simulink model "Commando07012014withscope"  (R2012b)
settings: Solver=ode5  StartTime=0.0  StopTime=inf  FixedStep=sample_time  RelTol=1e-3
InitFcn:
  | sample_time=0.005;%0.004;%0.0025;%0.02;
  | sample_time_Vicon = 0.005;
  | DeltaT = 0.02;
  | g = 9.81;
  | H0 = g%0.3165;
  | Kl = 1;
  | 
  | Q6_mass = 0.8;
  | 
  | Q6_Omega_r = 1.2; %for horizon ref
  | Q6_Zeta_r = 0.707; %for horizon ref
  | Q6_Omega_r_h = 2;%for vertical ref
  | Q6_Zeta_r_h = 0.7; %for vertical ref
  | 
  | 
  | Q6_Omega = 1.5; %for horizon control
  | Q6_Zeta = 0.507; %for horizon control
  | Q6_Omega_h= 2; %for vertical control
  | Q6_Zeta_h = 0.5; %for vertical control
  | 
  | 
  | Q6_acc_max = 5;%horizontal max acc
  | Q6_acc_max_h = 5;%horizontal max acc
  | 
  | omega_circle = 20*pi/180;
  | 
  | omega_h = 0.1;%Ascending speed
  | PI = pi;
  | Circle_R = 1.9;
  | 
  | 
  | MAX_Height = -2;
  | 
  | 
  | % for NN
  | n = 5;
  | r = 3;
  | n2 = 5;
  | NN_ST = 0.02;
  | 
  | GAMA_V = 6;
  | gama_V_e = 0.01;
  | 
  | GAMA_W = GAMA_V;
  | gama_W_e =0.01;
  | 
  | % deadzone
  | NN_Deadzone_Z = 0;
  | 
  | % inputs nomalizaton parameters
  | NN_Z_y_min = -3;
  | NN_Z_y_max = 0.5;
  | 
  | NN_Z_v_max = 8;
  | NN_Z_v_min = -NN_Z_v_max;
  | 
  | % alpha = 0.034;
  | alpha = 1;
  | % c_f = 0.0015;
  | c_f = 0.001;
  | ... (+1 lines)
libraries: X330_Control x20, simulink x10
(part 2 of 2)

== stateflow chart Commando07012014withscope/Subsystem/Trajectory Logic/ SF ==
  state Airborne
    state TakeOff
      du:		HoverThrottle = (H0 - HoverThrottle)*2*DeltaT + HoverThrottle ;
      PosDes_UAV1[2] = (-1.2 - PosDes_UAV1[2])*1*DeltaT + PosDes_UAV1[2] ;
      PosDes_UAV2[2] = (-1.2 - PosDes_UAV2[2])*1*DeltaT + PosDes_UAV2[2] ;
      PosDes_UAV3[2] = (-1.2 - PosDes_UAV3[2])*1*DeltaT + PosDes_UAV3[2] ;
      PosDes_UAV4[2] = (-1.2 - PosDes_UAV4[2])*1*DeltaT + PosDes_UAV4[2] ;
    state StartPoint
      state StartPoint_UAV1 [parallel]
        du:PosDes_UAV1[0] = (Circle_R*sin(0*PI/180 )- PosDes_UAV1[0])*1*DeltaT + PosDes_UAV1[0] ;
        PosDes_UAV1[1] = (Circle_R*cos(0*PI/180 )- PosDes_UAV1[1])*1*DeltaT + PosDes_UAV1[1] ;
        settings: executionOrder=1
      state StartPoint_UAV2 [parallel]
        du:PosDes_UAV2[0] = (Circle_R*sin(90*PI/180)-PosDes_UAV2[0])*0.5*DeltaT+PosDes_UAV2[0];
        PosDes_UAV2[1] = (Circle_R*cos(90*PI/180)-PosDes_UAV2[1])*0.5*DeltaT+PosDes_UAV2[1];
        settings: executionOrder=2
      state StartPoint_UAV3 [parallel]
        du:PosDes_UAV3[0] = (Circle_R*sin(180*PI/180)-PosDes_UAV3[0])*1*DeltaT + PosDes_UAV3[0];
        PosDes_UAV3[1] = (Circle_R*cos(180*PI/180)-PosDes_UAV3[1])*1*DeltaT+PosDes_UAV3[1];
        settings: executionOrder=3
      state test [parallel]
        settings: executionOrder=4
        state StartPoint_UAV4
          du:PosDes_UAV4[0] = (Circle_R*sin(270*PI/180)-PosDes_UAV4[0])*1*DeltaT+PosDes_UAV4[0];
          PosDes_UAV4[1] = (Circle_R*cos(270*PI/180)-PosDes_UAV4[1])*1*DeltaT+PosDes_UAV4[1];
        state Null
        (default) -> Null
        Null -> StartPoint_UAV4 : after(2,sec)
    state flyingcircle
      state Circle2D [parallel]
        du: PosDes_UAV1[0] = Circle_R*sin(0*PI/180 + T_circle*omega_circle);
        PosDes_UAV1[1] = Circle_R*cos(0*PI/180 + T_circle*omega_circle);
        PosDes_UAV1[2]= Pos_UAV5[2]-0.2;
        settings: executionOrder=1
      state Circle2D3 [parallel]
        du: PosDes_UAV4[0] = Circle_R*sin(270*PI/180 + T_circle*omega_circle);
        PosDes_UAV4[1] = Circle_R*cos(270*PI/180 + T_circle*omega_circle);
        PosDes_UAV4[2]= Pos_UAV5[2]-0.2;
        settings: executionOrder=2
      state Circle2D1 [parallel]
        du: PosDes_UAV2[0] = Circle_R*sin(90*PI/180 + T_circle*omega_circle);
        PosDes_UAV2[1] = Circle_R*cos(90*PI/180 + T_circle*omega_circle);
        PosDes_UAV2[2]= Pos_UAV5[2]-0.2;
        settings: executionOrder=3
      state T_Incr [parallel]
        du:   T_circle = T_circle + DeltaT;
        settings: executionOrder=4
      state Circle2D2 [parallel]
        du: PosDes_UAV3[0] = Circle_R*sin(180*PI/180 + T_circle*omega_circle);
        PosDes_UAV3[1] = Circle_R*cos(180*PI/180 + T_circle*omega_circle);
        PosDes_UAV3[2]= Pos_UAV5[2]-0.2;
        settings: executionOrder=5
    state flyingcircle1
      du:
      PosDes_UAV1[2] = (-2.7 - PosDes_UAV1[2])*0.5*DeltaT + PosDes_UAV1[2] ;
      PosDes_UAV2[2] = (-2.7 - PosDes_UAV2[2])*0.5*DeltaT + PosDes_UAV2[2] ;
      PosDes_UAV3[2] = (-2.7 - PosDes_UAV3[2])*0.5*DeltaT + PosDes_UAV3[2] ;
      PosDes_UAV4[2] = (-2.7 - PosDes_UAV4[2])*0.5*DeltaT + PosDes_UAV4[2] ;
    state flyingcircle2
      du:
      PosDes_UAV1[2] = (-1.2 - PosDes_UAV1[2])*1*DeltaT + PosDes_UAV1[2] ;
      PosDes_UAV2[2] = (-1.7 - PosDes_UAV2[2])*1*DeltaT + PosDes_UAV2[2] ;
      PosDes_UAV3[2] = (-2.2 - PosDes_UAV3[2])*1*DeltaT + PosDes_UAV3[2] ;
      PosDes_UAV4[2] = (-2.7 - PosDes_UAV4[2])*1*DeltaT + PosDes_UAV4[2] ;
    state endPoints
      du:
      PosDes_UAV1[2] = (-1.0 - PosDes_UAV1[2])*0.5*DeltaT + PosDes_UAV1[2] ;
      PosDes_UAV1[0]=(-2.0-PosDes_UAV1[0])*0.5*DeltaT+PosDes_UAV1[0];
      PosDes_UAV1[1]=(1.5-PosDes_UAV1[1])*0.5*DeltaT+PosDes_UAV1[1];
      PosDes_UAV2[2] = (-1.5 - PosDes_UAV2[2])*0.5*DeltaT + PosDes_UAV2[2] ;
      PosDes_UAV2[0]=(-2.0-PosDes_UAV2[0])*0.5*DeltaT+PosDes_UAV2[0];
      PosDes_UAV2[1]=(0.0-PosDes_UAV2[1])*0.5*DeltaT+PosDes_UAV2[1];
      PosDes_UAV3[2] = (-2.0 - PosDes_UAV3[2])*0.5*DeltaT + PosDes_UAV3[2] ;
      PosDes_UAV3[0]=(-2.0-PosDes_UAV3[0])*0.5*DeltaT+PosDes_UAV3[0];
      PosDes_UAV3[1]=(-1.5-PosDes_UAV3[1])*0.5*DeltaT+PosDes_UAV3[1];
      PosDes_UAV4[2] = (-2.5 - PosDes_UAV4[2])*0.5*DeltaT + PosDes_UAV4[2] ;
      PosDes_UAV4[0]=(-2.0-PosDes_UAV4[0])*0.5*DeltaT+PosDes_UAV4[0];
      PosDes_UAV4[1]=(-3.0-PosDes_UAV4[1])*0.5*DeltaT+PosDes_UAV4[1];
    state endPoints1
      du:
      PosDes_UAV1[2] = (-1.0 - PosDes_UAV1[2])*0.5*DeltaT + PosDes_UAV1[2] ;
      PosDes_UAV1[0]=(-2.0-PosDes_UAV1[0])*0.5*DeltaT+PosDes_UAV1[0];
      PosDes_UAV1[1]=(1.5-PosDes_UAV1[1])*0.5*DeltaT+PosDes_UAV1[1];
      PosDes_UAV2[2] = (-1.0 - PosDes_UAV2[2])*0.5*DeltaT + PosDes_UAV2[2] ;
      PosDes_UAV2[0]=(-2.0-PosDes_UAV2[0])*0.5*DeltaT+PosDes_UAV2[0];
      PosDes_UAV2[1]=(0.0-PosDes_UAV2[1])*0.5*DeltaT+PosDes_UAV2[1];
      PosDes_UAV3[2] = (-1.0 - PosDes_UAV3[2])*0.5*DeltaT + PosDes_UAV3[2] ;
      PosDes_UAV3[0]=(-2.0-PosDes_UAV3[0])*0.5*DeltaT+PosDes_UAV3[0];
      PosDes_UAV3[1]=(-1.5-PosDes_UAV3[1])*0.5*DeltaT+PosDes_UAV3[1];
      PosDes_UAV4[2] = (-1.0 - PosDes_UAV4[2])*0.5*DeltaT + PosDes_UAV4[2] ;
      PosDes_UAV4[0]=(-2.0-PosDes_UAV4[0])*0.5*DeltaT+PosDes_UAV4[0];
      PosDes_UAV4[1]=(-3.0-PosDes_UAV4[1])*0.5*DeltaT+PosDes_UAV4[1];
    (default) -> TakeOff : {	PosDes_UAV1 = Pos_UAV1;
        | 	PosDes_UAV2 = Pos_UAV2;
        | 	PosDes_UAV3 = Pos_UAV3;
        | 	PosDes_UAV4 = Pos_UAV4; }
    TakeOff -> StartPoint : after(3,sec)
    StartPoint -> flyingcircle : [abs(Pos_UAV4[0]-(-2))+abs(Pos_UAV4[1])<0.2]
        | {T_circle = 0.0, Light = 1;}
    flyingcircle -> flyingcircle1 : [RC[5]>0.5]
        | {Light=0;}
    flyingcircle1 -> flyingcircle2 : [abs(Pos_UAV5[0]-(-1))+abs(Pos_UAV5[1]-3.3)<0.3]
    flyingcircle2 -> endPoints : after (3,sec)
    endPoints -> endPoints1 : after (3,sec)
  state Landing
    state Decsending
      en:		PosDes_UAV1 = Pos_UAV1;	PosDes_UAV2 = Pos_UAV2;  PosDes_UAV3 = Pos_UAV3;
      PosDes_UAV4 = Pos_UAV4;
      du:		PosDes_UAV1[2] = (0 - PosDes_UAV1[2])*0.25*DeltaT + PosDes_UAV1[2] ;
      PosDes_UAV2[2] = (0 - PosDes_UAV2[2])*0.25*DeltaT + PosDes_UAV2[2] ;
      PosDes_UAV3[2] = (0 - PosDes_UAV3[2])*0.25*DeltaT + PosDes_UAV3[2] ;
      PosDes_UAV4[2] = (0 - PosDes_UAV4[2])*0.25*DeltaT + PosDes_UAV4[2] ;
    state CutThrottle
      du:		HoverThrottle = (0.0 - HoverThrottle)*3*DeltaT + HoverThrottle ;
    (default) -> Decsending
    Decsending -> (junction 288) : after(3,sec)
    (junction 288) -> CutThrottle : [Pos_UAV1[2] > -0.2]
  Landing -> Airborne : [RC[6] > 0.5]
      | {Light=0;}
  Airborne -> Landing : [RC[6] < -0.5]
      | {Light=0;}
  (default) -> Landing : {HoverThrottle=0.0, Light = 0;}
  data: HoverThrottle output double size=1; PosDes_UAV1 output double size=4; PosDes_UAV2 output double size=4; PosDes_UAV3 output double size=4; RC input size=8; Pos_UAV1 input size=4; DeltaT parameter size=1; H0 parameter size=1; Kl parameter size=1; T_circle local double size=1; omega_circle parameter size=1; PI parameter size=1; omega_h parameter; Circle_R parameter size=1; MAX_Height parameter size=1; Pos_UAV2 input size=4; Pos_UAV3 input size=4; Pos_UAV4 input size=4; Pos_UAV5 input size=4; PosDes_UAV4 output double size=4; Light output double size=1 =0
